simulink model "ur_data_record"  (R2024a)
settings: Solver=FixedStepAuto  StartTime=0.0  StopTime=inf  FixedStep=0.03  RelTol=1e-3
libraries: ros2lib x18
settings Model: Creator=ASUS  LastModifiedBy=echoz

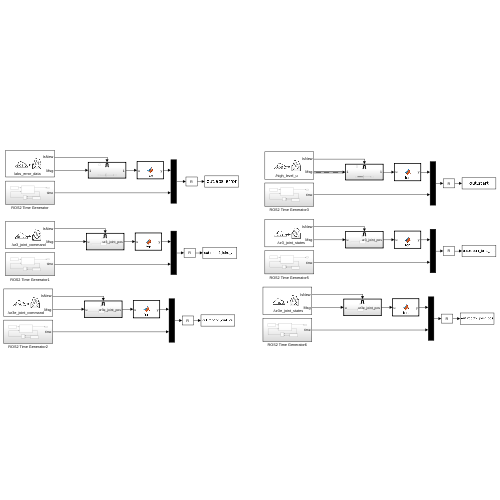
[thumbnail: Simulink's stored preview of the top-level diagram]
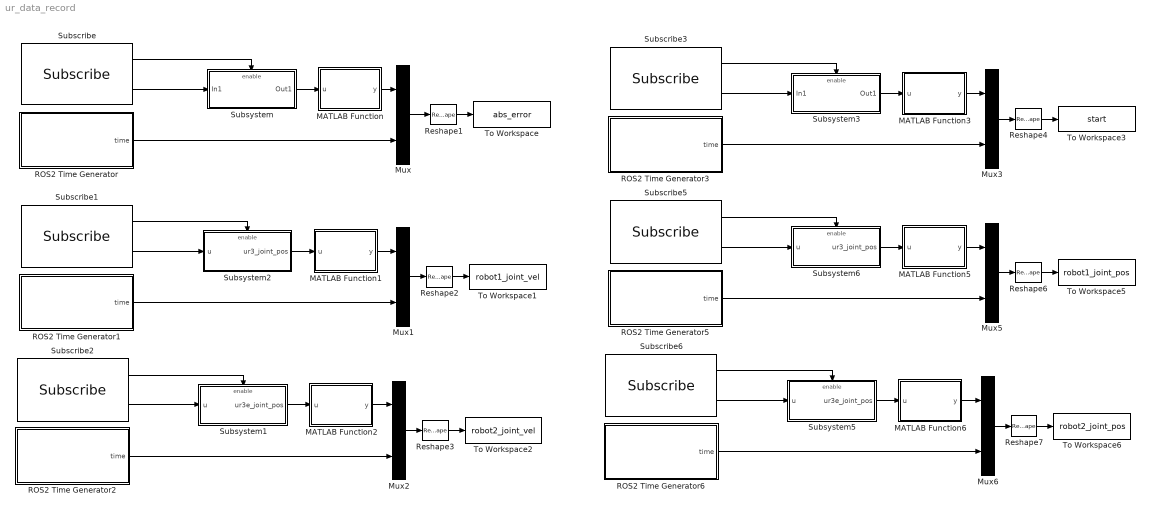
== system ur_data_record ==
  MATLAB Function : MATLAB Function  TreatAsAtomicUnit=on
  MATLAB Function1 : MATLAB Function  TreatAsAtomicUnit=on
  MATLAB Function2 : MATLAB Function  TreatAsAtomicUnit=on
  MATLAB Function3 : MATLAB Function  TreatAsAtomicUnit=on
  MATLAB Function5 : MATLAB Function  TreatAsAtomicUnit=on
  MATLAB Function6 : MATLAB Function  TreatAsAtomicUnit=on
  Mux{,1..3,5..6} (6 alike) : Mux  Inputs=2
  ROS2 Time Generator : Subsystem
  ROS2 Time Generator1 : Subsystem
  ROS2 Time Generator2 : Subsystem
  ROS2 Time Generator3 : Subsystem
  ROS2 Time Generator5 : Subsystem
  ROS2 Time Generator6 : Subsystem
  Reshape1 : Reshape  OutputDimensionality=Customize  OutputDimensions=[9]
  Reshape{2..3,6..7} (4 alike) : Reshape  OutputDimensionality=Customize  OutputDimensions=[7]
  Reshape4 : Reshape  OutputDimensionality=Customize  OutputDimensions=[2]
  Subscribe : ros2lib/Subscribe  topicSource=Select from ROS network  topic=/abs_error_data  messageType=std_msgs/Float64MultiArray  sampleTime=-1  QOSHistory=Keep last  QOSDepth=1  QOSReliability=Reliable  QOSDurability=Volatile  QOSDeadline=Inf  QOSLifespan=Inf  QOSLiveliness=Automatic  QOSLeaseDuration=Inf  QOSAvoidROSNamespaceConventions=off
  Subscribe1 : ros2lib/Subscribe  topicSource=Select from ROS network  topic=/ur3_joint_command  messageType=sensor_msgs/JointState  sampleTime=-1  QOSHistory=Keep last  QOSDepth=1  QOSReliability=Reliable  QOSDurability=Volatile  QOSDeadline=Inf  QOSLifespan=Inf  QOSLiveliness=Automatic  QOSLeaseDuration=Inf  QOSAvoidROSNamespaceConventions=off
  Subscribe2 : ros2lib/Subscribe  topicSource=Select from ROS network  topic=/ur3e_joint_command  messageType=sensor_msgs/JointState  sampleTime=-1  QOSHistory=Keep last  QOSDepth=1  QOSReliability=Reliable  QOSDurability=Volatile  QOSDeadline=Inf  QOSLifespan=Inf  QOSLiveliness=Automatic  QOSLeaseDuration=Inf  QOSAvoidROSNamespaceConventions=off
  Subscribe3 : ros2lib/Subscribe  topicSource=Select from ROS network  topic=/high_level_u  messageType=std_msgs/Float64MultiArray  sampleTime=-1  QOSHistory=Keep last  QOSDepth=1  QOSReliability=Reliable  QOSDurability=Volatile  QOSDeadline=Inf  QOSLifespan=Inf  QOSLiveliness=Automatic  QOSLeaseDuration=Inf  QOSAvoidROSNamespaceConventions=off
  Subscribe5 : ros2lib/Subscribe  topicSource=Select from ROS network  topic=/ur3_joint_states  messageType=sensor_msgs/JointState  sampleTime=-1  QOSHistory=Keep last  QOSDepth=1  QOSReliability=Reliable  QOSDurability=Volatile  QOSDeadline=Inf  QOSLifespan=Inf  QOSLiveliness=Automatic  QOSLeaseDuration=Inf  QOSAvoidROSNamespaceConventions=off
  Subscribe6 : ros2lib/Subscribe  topicSource=Select from ROS network  topic=/ur3e_joint_states  messageType=sensor_msgs/JointState  sampleTime=-1  QOSHistory=Keep last  QOSDepth=1  QOSReliability=Reliable  QOSDurability=Volatile  QOSDeadline=Inf  QOSLifespan=Inf  QOSLiveliness=Automatic  QOSLeaseDuration=Inf  QOSAvoidROSNamespaceConventions=off
  Subsystem : Subsystem
  Subsystem1 : Subsystem
  Subsystem2 : Subsystem
  Subsystem3 : Subsystem
  Subsystem5 : Subsystem
  Subsystem6 : Subsystem
  To Workspace : ToWorkspace  VariableName=abs_error  SaveFormat=Timeseries  SampleTime=-1
  To Workspace1 : ToWorkspace  VariableName=robot1_joint_vel  SaveFormat=Timeseries  SampleTime=-1
  To Workspace2 : ToWorkspace  VariableName=robot2_joint_vel  SaveFormat=Timeseries  SampleTime=-1
  To Workspace3 : ToWorkspace  VariableName=start  SaveFormat=Timeseries  SampleTime=-1
  To Workspace5 : ToWorkspace  VariableName=robot1_joint_pos  SaveFormat=Timeseries  SampleTime=-1
  To Workspace6 : ToWorkspace  VariableName=robot2_joint_pos  SaveFormat=Timeseries  SampleTime=-1
  wires:
  Subscribe/2 -> Subsystem/1(In1)
  Subscribe/1 -> Subsystem/Enable
  Mux/1 -> Reshape1/1
  ROS2 Time Generator/1(time) -> Mux/2
  Reshape1/1 -> To Workspace/1
  Subsystem/1(Out1) -> MATLAB Function/1(u)
  MATLAB Function/1(y) -> Mux/1
  Subscribe1/2 -> Subsystem2/1(u)
  Subscribe1/1 -> Subsystem2/Enable
  Subsystem2/1(ur3_joint_pos) -> MATLAB Function1/1(u)
  MATLAB Function1/1(y) -> Mux1/1
  ROS2 Time Generator1/1(time) -> Mux1/2
  Mux1/1 -> Reshape2/1
  Reshape2/1 -> To Workspace1/1
  Mux2/1 -> Reshape3/1
  ROS2 Time Generator2/1(time) -> Mux2/2
  Subscribe2/2 -> Subsystem1/1(u)
  MATLAB Function2/1(y) -> Mux2/1
  Subsystem1/1(ur3e_joint_pos) -> MATLAB Function2/1(u)
  Subscribe2/1 -> Subsystem1/Enable
  Reshape3/1 -> To Workspace2/1
  ROS2 Time Generator6/1(time) -> Mux6/2
  ROS2 Time Generator5/1(time) -> Mux5/2
  Reshape7/1 -> To Workspace6/1
  Subscribe6/1 -> Subsystem5/Enable
  Subsystem6/1(ur3_joint_pos) -> MATLAB Function5/1(u)
  Mux6/1 -> Reshape7/1
  MATLAB Function5/1(y) -> Mux5/1
  Subscribe5/1 -> Subsystem6/Enable
  Subsystem5/1(ur3e_joint_pos) -> MATLAB Function6/1(u)
  MATLAB Function6/1(y) -> Mux6/1
  Subscribe5/2 -> Subsystem6/1(u)
  Subscribe6/2 -> Subsystem5/1(u)
  Mux5/1 -> Reshape6/1
  Reshape6/1 -> To Workspace5/1
  Mux3/1 -> Reshape4/1
  Subscribe3/2 -> Subsystem3/1(In1)
  Reshape4/1 -> To Workspace3/1
  MATLAB Function3/1(y) -> Mux3/1
  ROS2 Time Generator3/1(time) -> Mux3/2
  Subsystem3/1(Out1) -> MATLAB Function3/1(u)
  Subscribe3/1 -> Subsystem3/Enable

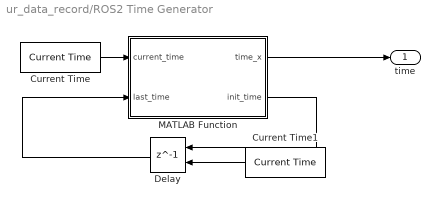
== system ur_data_record/ROS2 Time Generator ==
  Current Time : ros2lib/Current Time  OutputFormat=double  SampleTime=-1  ModelName=ur_data_record
      settings: LibrarySourceBlock=roslib/ROS 2/Current Time
  Current Time1 : ros2lib/Current Time  OutputFormat=double  SampleTime=-1  ModelName=ur_data_record
      settings: LibrarySourceBlock=roslib/ROS 2/Current Time
  Delay : Delay  DelayLength=1  InitialConditionSource=Input port
      settings: InputPortMap=u0,p4
  MATLAB Function : MATLAB Function  TreatAsAtomicUnit=on
  time : Outport
  wires:
  Delay/1 -> MATLAB Function/2(last_time)
  Current Time1/1 -> Delay/2
  MATLAB Function/2(init_time) -> Delay/1
  Current Time/1 -> MATLAB Function/1(current_time)
  MATLAB Function/1(time_x) -> time/1

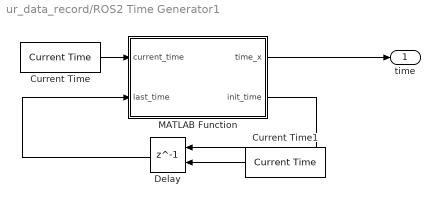
== system ur_data_record/ROS2 Time Generator1 ==
  Current Time : ros2lib/Current Time  OutputFormat=double  SampleTime=-1  ModelName=ur_data_record
      settings: LibrarySourceBlock=roslib/ROS 2/Current Time
  Current Time1 : ros2lib/Current Time  OutputFormat=double  SampleTime=-1  ModelName=ur_data_record
      settings: LibrarySourceBlock=roslib/ROS 2/Current Time
  Delay : Delay  DelayLength=1  InitialConditionSource=Input port
      settings: InputPortMap=u0,p4
  MATLAB Function : MATLAB Function  TreatAsAtomicUnit=on
  time : Outport
  wires:
  Delay/1 -> MATLAB Function/2(last_time)
  Current Time1/1 -> Delay/2
  MATLAB Function/2(init_time) -> Delay/1
  Current Time/1 -> MATLAB Function/1(current_time)
  MATLAB Function/1(time_x) -> time/1

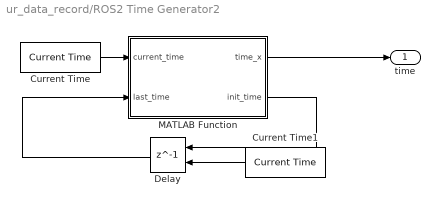
== system ur_data_record/ROS2 Time Generator2 ==
  Current Time : ros2lib/Current Time  OutputFormat=double  SampleTime=-1  ModelName=ur_data_record
      settings: LibrarySourceBlock=roslib/ROS 2/Current Time
  Current Time1 : ros2lib/Current Time  OutputFormat=double  SampleTime=-1  ModelName=ur_data_record
      settings: LibrarySourceBlock=roslib/ROS 2/Current Time
  Delay : Delay  DelayLength=1  InitialConditionSource=Input port
      settings: InputPortMap=u0,p4
  MATLAB Function : MATLAB Function  TreatAsAtomicUnit=on
  time : Outport
  wires:
  Delay/1 -> MATLAB Function/2(last_time)
  Current Time1/1 -> Delay/2
  MATLAB Function/2(init_time) -> Delay/1
  Current Time/1 -> MATLAB Function/1(current_time)
  MATLAB Function/1(time_x) -> time/1

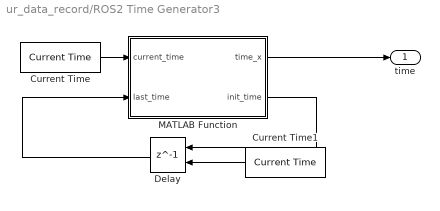
== system ur_data_record/ROS2 Time Generator3 ==
  Current Time : ros2lib/Current Time  OutputFormat=double  SampleTime=-1  ModelName=ur_data_record
      settings: LibrarySourceBlock=roslib/ROS 2/Current Time
  Current Time1 : ros2lib/Current Time  OutputFormat=double  SampleTime=-1  ModelName=ur_data_record
      settings: LibrarySourceBlock=roslib/ROS 2/Current Time
  Delay : Delay  DelayLength=1  InitialConditionSource=Input port
      settings: InputPortMap=u0,p4
  MATLAB Function : MATLAB Function  TreatAsAtomicUnit=on
  time : Outport
  wires:
  Delay/1 -> MATLAB Function/2(last_time)
  Current Time1/1 -> Delay/2
  MATLAB Function/2(init_time) -> Delay/1
  Current Time/1 -> MATLAB Function/1(current_time)
  MATLAB Function/1(time_x) -> time/1

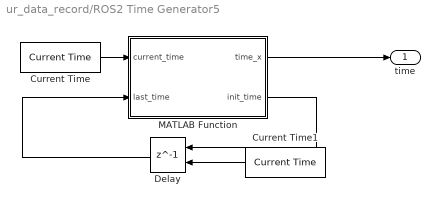
== system ur_data_record/ROS2 Time Generator5 ==
  Current Time : ros2lib/Current Time  OutputFormat=double  SampleTime=-1  ModelName=ur_data_record
      settings: LibrarySourceBlock=roslib/ROS 2/Current Time
  Current Time1 : ros2lib/Current Time  OutputFormat=double  SampleTime=-1  ModelName=ur_data_record
      settings: LibrarySourceBlock=roslib/ROS 2/Current Time
  Delay : Delay  DelayLength=1  InitialConditionSource=Input port
      settings: InputPortMap=u0,p4
  MATLAB Function : MATLAB Function  TreatAsAtomicUnit=on
  time : Outport
  wires:
  Delay/1 -> MATLAB Function/2(last_time)
  Current Time1/1 -> Delay/2
  MATLAB Function/2(init_time) -> Delay/1
  Current Time/1 -> MATLAB Function/1(current_time)
  MATLAB Function/1(time_x) -> time/1

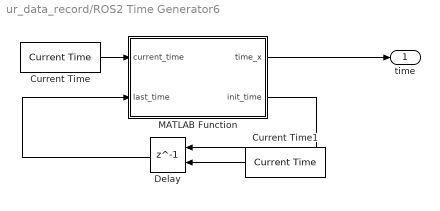
== system ur_data_record/ROS2 Time Generator6 ==
  Current Time : ros2lib/Current Time  OutputFormat=double  SampleTime=-1  ModelName=ur_data_record
      settings: LibrarySourceBlock=roslib/ROS 2/Current Time
  Current Time1 : ros2lib/Current Time  OutputFormat=double  SampleTime=-1  ModelName=ur_data_record
      settings: LibrarySourceBlock=roslib/ROS 2/Current Time
  Delay : Delay  DelayLength=1  InitialConditionSource=Input port
      settings: InputPortMap=u0,p4
  MATLAB Function : MATLAB Function  TreatAsAtomicUnit=on
  time : Outport
  wires:
  Delay/1 -> MATLAB Function/2(last_time)
  Current Time1/1 -> Delay/2
  MATLAB Function/2(init_time) -> Delay/1
  Current Time/1 -> MATLAB Function/1(current_time)
  MATLAB Function/1(time_x) -> time/1

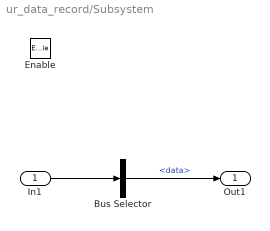
== system ur_data_record/Subsystem ==
  In1 : Inport
  Enable : EnablePort
  Bus Selector : BusSelector  OutputSignals=data
  Out1 : Outport
  wires:
  In1/1 -> Bus Selector/1
  Bus Selector/1 -> Out1/1  "<data>"

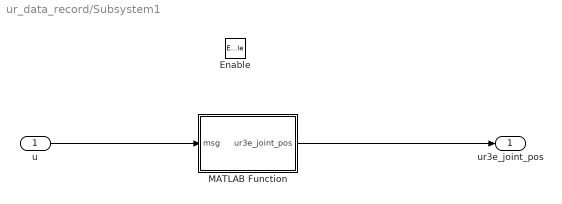
== system ur_data_record/Subsystem1 ==
  u : Inport
  Enable : EnablePort
  MATLAB Function : MATLAB Function  TreatAsAtomicUnit=on
  ur3e_joint_pos : Outport
  wires:
  u/1 -> MATLAB Function/1(msg)
  MATLAB Function/1(ur3e_joint_pos) -> ur3e_joint_pos/1

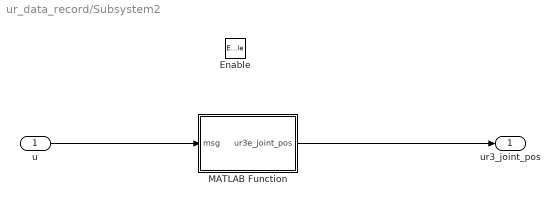
== system ur_data_record/Subsystem2 ==
  u : Inport
  Enable : EnablePort
  MATLAB Function : MATLAB Function  TreatAsAtomicUnit=on
  ur3_joint_pos : Outport
  wires:
  u/1 -> MATLAB Function/1(msg)
  MATLAB Function/1(ur3e_joint_pos) -> ur3_joint_pos/1

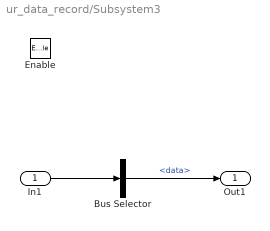
== system ur_data_record/Subsystem3 ==
  In1 : Inport
  Enable : EnablePort
  Bus Selector : BusSelector  OutputSignals=data
  Out1 : Outport
  wires:
  In1/1 -> Bus Selector/1
  Bus Selector/1 -> Out1/1  "<data>"

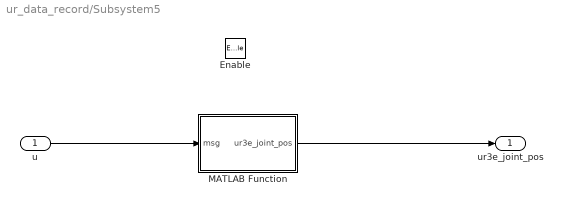
== system ur_data_record/Subsystem5 ==
  u : Inport
  Enable : EnablePort
  MATLAB Function : MATLAB Function  TreatAsAtomicUnit=on
  ur3e_joint_pos : Outport
  wires:
  u/1 -> MATLAB Function/1(msg)
  MATLAB Function/1(ur3e_joint_pos) -> ur3e_joint_pos/1

== system ur_data_record/Subsystem6 ==
  u : Inport
  Enable : EnablePort
  MATLAB Function : MATLAB Function  TreatAsAtomicUnit=on
  ur3_joint_pos : Outport
  wires:
  u/1 -> MATLAB Function/1(msg)
  MATLAB Function/1(ur3e_joint_pos) -> ur3_joint_pos/1

== matlab function ur_data_record/Subsystem5/MATLAB Function ==
  data: msg input; ur3e_joint_pos output
function ur3e_joint_pos = fcn(msg)
ur3e_joint_pos = msg.position(1:6);

== matlab function ur_data_record/Subsystem6/MATLAB Function ==
  data: msg input; ur3e_joint_pos output
function ur3e_joint_pos = fcn(msg)
ur3e_joint_pos = msg.position(1:6);

== matlab function ur_data_record/Subsystem2/MATLAB Function ==
  data: msg input; ur3e_joint_pos output
function ur3e_joint_pos = fcn(msg)
ur3e_joint_pos = msg.velocity(1:6);

== matlab function ur_data_record/ROS2 Time Generator/MATLAB Function ==
  data: current_time input; last_time input; time_x output; init_time output
function [time_x,init_time] = fcn(current_time, last_time)
init_time = last_time;
time_x = current_time-last_time;

== matlab function ur_data_record/MATLAB Function ==
  data: u input; y output
function y = fcn(u)

y = u(1:8);

== matlab function ur_data_record/ROS2 Time Generator1/MATLAB Function ==
  data: current_time input; last_time input; time_x output; init_time output
function [time_x,init_time] = fcn(current_time, last_time)
init_time = last_time;
time_x = current_time-last_time;

== matlab function ur_data_record/MATLAB Function2 ==
  data: u input; y output
function y = fcn(u)

y = u(1:6);

== matlab function ur_data_record/ROS2 Time Generator2/MATLAB Function ==
  data: current_time input; last_time input; time_x output; init_time output
function [time_x,init_time] = fcn(current_time, last_time)
init_time = last_time;
time_x = current_time-last_time;

== matlab function ur_data_record/Subsystem1/MATLAB Function ==
  data: msg input; ur3e_joint_pos output
function ur3e_joint_pos = fcn(msg)
ur3e_joint_pos = msg.velocity(1:6);

== matlab function ur_data_record/MATLAB Function3 ==
  data: u input; y output
function y = fcn(u)

y = u(1);

== matlab function ur_data_record/ROS2 Time Generator3/MATLAB Function ==
  data: current_time input; last_time input; time_x output; init_time output
function [time_x,init_time] = fcn(current_time, last_time)
init_time = last_time;
time_x = current_time-last_time;

== matlab function ur_data_record/MATLAB Function5 ==
  data: u input; y output
function y = fcn(u)

y = u(1:6);

== matlab function ur_data_record/MATLAB Function6 ==
  data: u input; y output
function y = fcn(u)

y = u(1:6);

== matlab function ur_data_record/ROS2 Time Generator5/MATLAB Function ==
  data: current_time input; last_time input; time_x output; init_time output
function [time_x,init_time] = fcn(current_time, last_time)
init_time = last_time;
time_x = current_time-last_time;

== matlab function ur_data_record/MATLAB Function1 ==
  data: u input; y output
function y = fcn(u)

y = u(1:6);

== matlab function ur_data_record/ROS2 Time Generator6/MATLAB Function ==
  data: current_time input; last_time input; time_x output; init_time output
function [time_x,init_time] = fcn(current_time, last_time)
init_time = last_time;
time_x = current_time-last_time;
